simulink model "exampleEnthalpy"  (Simulink 7.6)
settings: Solver=ode45  StartTime=0.0  StopTime=10.0  RelTol=1e-3
libraries: carnot x4
settings Model: Creator=drhf  LastModifiedBy=drhf

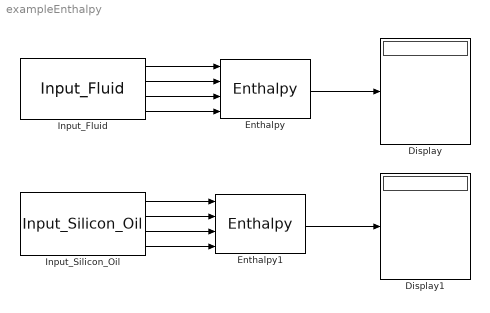
== system exampleEnthalpy ==
  Display : Display
  Display1 : Display
  Enthalpy : carnot/Basic/Material_Properties/Enthalpy  SystemSampleTime=-1
  Enthalpy1 : carnot/Basic/Material_Properties/Enthalpy  SystemSampleTime=-1
  Input_Fluid : carnot/Basic/Material_Properties/Input_Fluid  SystemSampleTime=-1  fluid=water  T=[10:10:50]  p=1e5  x=0.005
  Input_Silicon_Oil : carnot/Basic/Material_Properties/Input_Silicon_Oil  SystemSampleTime=-1  T=[10:10:50]  p=1e5
  wires:
  Input_Fluid/1 -> Enthalpy/1
  Input_Fluid/2 -> Enthalpy/2
  Input_Fluid/3 -> Enthalpy/3
  Input_Fluid/4 -> Enthalpy/4
  Enthalpy/1 -> Display/1
  Input_Silicon_Oil/1 -> Enthalpy1/1
  Input_Silicon_Oil/2 -> Enthalpy1/2
  Input_Silicon_Oil/3 -> Enthalpy1/3
  Input_Silicon_Oil/4 -> Enthalpy1/4
  Enthalpy1/1 -> Display1/1
